simulink model "Quadrotor"  (R2013b)
settings: Solver=ode45  StartTime=0.0  StopTime=10.0  MaxStep=0.1  RelTol=1e-3
InitFcn:
  | parameters;
  | [b, d] = Bemt();
values from neighbouring files (symbols this model uses):
  attitudeInit = [0;0;0]    [parameters.m]
  b = (sigma*Cla/8-lambdaV)    [Bemt.m]
  g = 9.81    [parameters.m]
  I = diag([0.0086,0.0086,0.0172])    [parameters.m]
  Iprop = 12*10^-6    (= 1.2e-05)    [parameters.m]
  Kmot = 1/(1900/60*2*pi)    (= 0.00502594557132)    [parameters.m]
  L = 0.225    [parameters.m]
  m = 0.58    [parameters.m]
  MotorSpeedInit = [300;300;300;300]    [parameters.m]
  omegaInit = [0;0;0]    [parameters.m]
  posInit = [0;0;0]    [parameters.m]
  Rmot = 0.128    [parameters.m]
  velInit = [0;0;0]    [parameters.m]
undefined symbols (not defined in the file or in its folder): d
settings Model: Creator=rudink  LastModifiedBy=rudink
settings DebuggingCC: StateNameClashWarn=warning

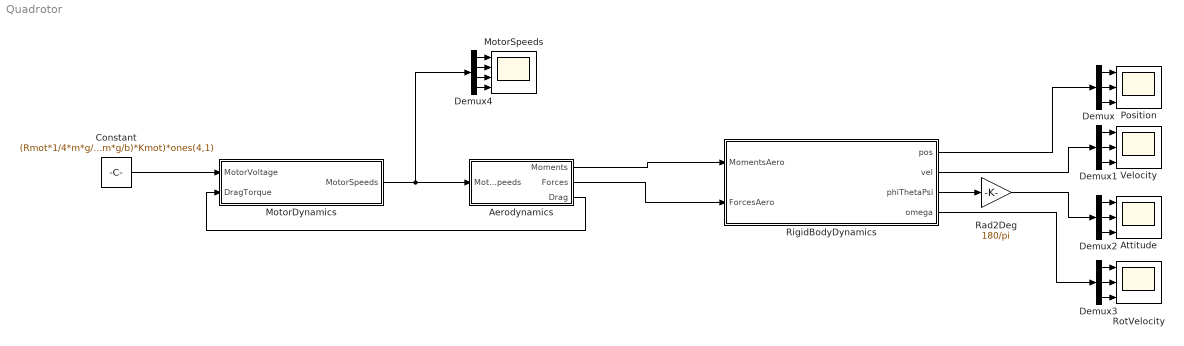
== system Quadrotor ==
  Aerodynamics : Subsystem
  Attitude : Scope  NumInputPorts=3
      settings: YMin=-5~-5~-5  YMax=5~5~5  SaveName=ScopeData2  MaxDataPoints=10000
  Constant : Constant  Value=(Rmot*1/4*m*g/b*d/Kmot+sqrt(1/4*m*g/b)*Kmot)*ones(4,1)
  Demux{,1..3} (4 alike) : Demux  Outputs=3
  Demux4 : Demux
  MotorDynamics : Subsystem
  MotorSpeeds : Scope  NumInputPorts=4
      settings: YMin=-5~-5~-5~-5  YMax=5~5~5~5  SaveName=ScopeData4  MaxDataPoints=10000
  Position : Scope  NumInputPorts=3
      settings: YMin=-5~-5~-5  YMax=5~5~5  MaxDataPoints=10000
  Rad2Deg : Gain  Gain=180/pi
  RigidBodyDynamics : Subsystem
  RotVelocity : Scope  NumInputPorts=3
      settings: YMin=-5~-5~-5  YMax=5~5~5  SaveName=ScopeData3  MaxDataPoints=10000
  Velocity : Scope  NumInputPorts=3
      settings: YMin=-5~-5~-5  YMax=5~5~5  MaxDataPoints=10000
  wires:
  Demux/2 -> Position/2
  Demux/3 -> Position/3
  Demux/1 -> Position/1
  RigidBodyDynamics/1(pos) -> Demux/1
  Demux1/2 -> Velocity/2
  Demux1/3 -> Velocity/3
  Demux1/1 -> Velocity/1
  Demux2/2 -> Attitude/2
  Demux2/3 -> Attitude/3
  Demux2/1 -> Attitude/1
  Demux3/2 -> RotVelocity/2
  Demux3/3 -> RotVelocity/3
  Demux3/1 -> RotVelocity/1
  RigidBodyDynamics/2(vel) -> Demux1/1
  RigidBodyDynamics/3(phiThetaPsi) -> Rad2Deg/1
  RigidBodyDynamics/4(omega) -> Demux3/1
  Aerodynamics/2(Forces) -> RigidBodyDynamics/2(ForcesAero)
  Aerodynamics/1(Moments) -> RigidBodyDynamics/1(MomentsAero)
  Rad2Deg/1 -> Demux2/1
  MotorDynamics/1(MotorSpeeds) -> Demux4/1, Aerodynamics/1(MotorSpeeds)
  Aerodynamics/3(Drag) -> MotorDynamics/2(DragTorque)
  Constant/1 -> MotorDynamics/1(MotorVoltage)
  Demux4/2 -> MotorSpeeds/2
  Demux4/1 -> MotorSpeeds/1
  Demux4/3 -> MotorSpeeds/3
  Demux4/4 -> MotorSpeeds/4

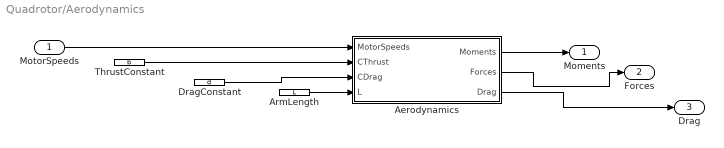
== system Quadrotor/Aerodynamics ==
  MotorSpeeds : Inport
  Aerodynamics : MATLAB Function  TreatAsAtomicUnit=on
  ArmLength : Constant  Value=L
  DragConstant : Constant  Value=d
  ThrustConstant : Constant  Value=b
  Moments : Outport
  Forces : Outport  Port=2
  Drag : Outport  Port=3
  wires:
  Aerodynamics/1(Moments) -> Moments/1
  Aerodynamics/2(Forces) -> Forces/1
  MotorSpeeds/1 -> Aerodynamics/1(MotorSpeeds)
  ThrustConstant/1 -> Aerodynamics/2(CThrust)
  DragConstant/1 -> Aerodynamics/3(CDrag)
  ArmLength/1 -> Aerodynamics/4(L)
  Aerodynamics/3(Drag) -> Drag/1

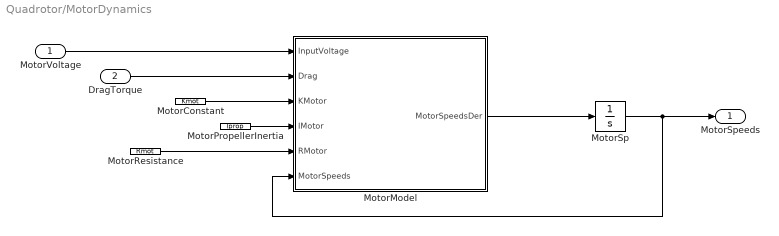
== system Quadrotor/MotorDynamics ==
  MotorVoltage : Inport
  DragTorque : Inport  Port=2
  MotorConstant : Constant  Value=Kmot
  MotorModel : MATLAB Function  TreatAsAtomicUnit=on
  MotorPropellerInertia : Constant  Value=Iprop
  MotorResistance : Constant  Value=Rmot
  MotorSp : Integrator  InitialCondition=MotorSpeedInit
  MotorSpeeds : Outport
  wires:
  MotorVoltage/1 -> MotorModel/1(InputVoltage)
  DragTorque/1 -> MotorModel/2(Drag)
  MotorModel/1(MotorSpeedsDer) -> MotorSp/1
  MotorSp/1 -> MotorModel/6(MotorSpeeds), MotorSpeeds/1
  MotorConstant/1 -> MotorModel/3(KMotor)
  MotorPropellerInertia/1 -> MotorModel/4(IMotor)
  MotorResistance/1 -> MotorModel/5(RMotor)

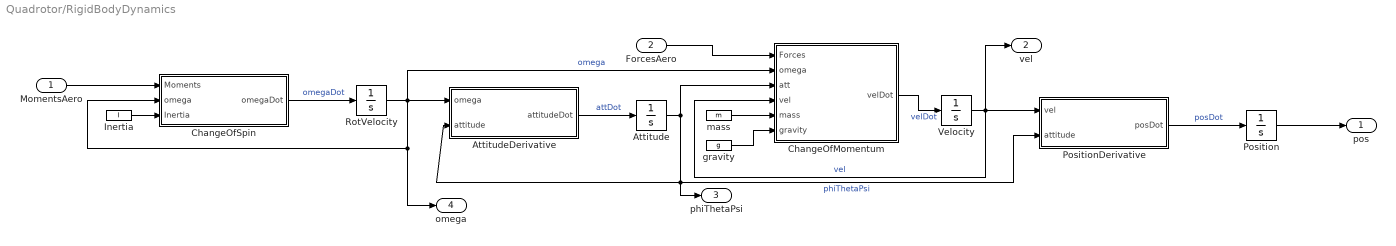
== system Quadrotor/RigidBodyDynamics ==
  MomentsAero : Inport
  ForcesAero : Inport  Port=2
  Attitude : Integrator  InitialCondition=attitudeInit
  AttitudeDerivative : MATLAB Function  TreatAsAtomicUnit=on
  ChangeOfMomentum : MATLAB Function  TreatAsAtomicUnit=on
  ChangeOfSpin : MATLAB Function  TreatAsAtomicUnit=on
  Inertia : Constant  Value=I
  Position : Integrator  InitialCondition=posInit
  PositionDerivative : MATLAB Function  TreatAsAtomicUnit=on
  RotVelocity : Integrator  InitialCondition=omegaInit
  Velocity : Integrator  InitialCondition=velInit
  gravity : Constant  Value=g
  mass : Constant  Value=m
  pos : Outport
  vel : Outport  Port=2
  phiThetaPsi : Outport  Port=3
  omega : Outport  Port=4
  wires:
  MomentsAero/1 -> ChangeOfSpin/1(Moments)
  ChangeOfSpin/1(omegaDot) -> RotVelocity/1  "omegaDot"
  RotVelocity/1 -> ChangeOfMomentum/2(omega), AttitudeDerivative/1(omega), omega/1, ChangeOfSpin/2(omega)  "omega"
  AttitudeDerivative/1(attitudeDot) -> Attitude/1  "attDot"
  Attitude/1 -> ChangeOfMomentum/3(att), phiThetaPsi/1, PositionDerivative/2(attitude), AttitudeDerivative/2(attitude)  "phiThetaPsi"
  ChangeOfMomentum/1(velDot) -> Velocity/1  "velDot"
  Velocity/1 -> vel/1, PositionDerivative/1(vel), ChangeOfMomentum/4(vel)  "vel"
  ForcesAero/1 -> ChangeOfMomentum/1(Forces)
  PositionDerivative/1(posDot) -> Position/1  "posDot"
  Position/1 -> pos/1
  Inertia/1 -> ChangeOfSpin/3(Inertia)
  mass/1 -> ChangeOfMomentum/5(mass)
  gravity/1 -> ChangeOfMomentum/6(gravity)

== matlab function Quadrotor/RigidBodyDynamics/AttitudeDerivative ==
  data: omega input; attitude input; attitudeDot output
function attitudeDot = fcn(omega, attitude)
%#codegen
phi = attitude(1);
theta = attitude(2);

% Calculate the inverse of the jacobian relating the taith-Brian angle to
% body rates
Jinv = [1 sin(phi)*tan(theta) cos(phi)*tan(theta);...
        0            cos(phi)           -sin(phi);...
        0 sin(phi)/cos(theta) cos(phi)/cos(theta)];

attitudeDot = Jinv*omega;

== matlab function Quadrotor/RigidBodyDynamics/ChangeOfSpin ==
  data: Moments input; omegaDot output; omega input; Inertia input
function omegaDot = fcn(Moments, omega, Inertia)
%#codegen

omegaDot = Inertia^(-1)*(Moments-cross(omega,Inertia*omega));

== matlab function Quadrotor/RigidBodyDynamics/ChangeOfMomentum ==
  data: Forces input; velDot output; omega input; att input; vel input; mass input; gravity input
function velDot = fcn(Forces, omega, att, vel, mass, gravity)
%#codegen
phi = att(1);
theta = att(2);

% Calculate the gravitational acceleration
g = [-sin(theta);...
      sin(phi)*cos(theta);...
      cos(phi)*cos(theta)]*gravity;
  
% Calculate the derivative of the velocity  
velDot = 1/mass*Forces+g-cross(omega,vel);

== matlab function Quadrotor/RigidBodyDynamics/PositionDerivative ==
  data: vel input; attitude input; posDot output
function posDot = fcn(vel, attitude)
%#codegen
phi = attitude(1);
theta = attitude(2);
psi = attitude(3);

% Calculate the rotational Matrix
R = [cos(theta)*cos(psi) sin(phi)*sin(theta)*cos(psi)-cos(phi)*sin(psi) cos(phi)*sin(theta)*cos(psi)+sin(phi)*sin(psi);...
     cos(theta)*sin(psi) sin(phi)*sin(theta)*sin(psi)+cos(phi)*cos(psi) cos(phi)*sin(theta)*sin(psi)-sin(phi)*cos(psi);...
             -sin(theta)                            sin(phi)*cos(theta)                            cos(phi)*cos(theta)];

posDot = R*vel;

== matlab function Quadrotor/Aerodynamics/Aerodynamics ==
  data: MotorSpeeds input; Moments output; Forces output; CThrust input; CDrag input; L input; Drag output
function [Moments, Forces, Drag] = fcn(MotorSpeeds,CThrust,CDrag,L)
%#codegen
Drag = CDrag*MotorSpeeds.^2;
Forces = [0;0;-sum(CThrust*MotorSpeeds.^2)];
Moments = [L*CThrust*(MotorSpeeds(4).^2-MotorSpeeds(2).^2);...
           L*CThrust*(MotorSpeeds(1).^2-MotorSpeeds(3).^2);...
           Drag(1)-Drag(2)+Drag(3)-Drag(4)];

== matlab function Quadrotor/MotorDynamics/MotorModel ==
  data: InputVoltage input; Drag input; KMotor input; IMotor input; RMotor input; MotorSpeeds input; MotorSpeedsDer output
function MotorSpeedsDer = fcn(InputVoltage,Drag,KMotor,IMotor,RMotor, MotorSpeeds)
%#codegen

% Calculate the Current
Uind = KMotor*MotorSpeeds;
i = (InputVoltage-Uind)/RMotor;

% Calculate the derivative of the motorspeed
MotorSpeedsDer = (KMotor*i-Drag)/IMotor;
